simulink model "VarLoad"  (R2016a)
settings: Solver=ode23t  StartTime=0.0  StopTime=6  FixedStep=t_PWM/10  MaxStep=2e-6  RelTol=2e-4
values from neighbouring files (symbols this model uses):
  C1 = t_PWM * (N*Impp)*0.1/ (8 * (N*Vmpp)*0.0001)    [SolarPanelModel.m]
  C2 = (N*Vo) * t_PWM/ (Load * (N*Vo)*0.001)    [SolarPanelModel.m]
  Isc = G/ Gr * (Iscr + miu_Isc*(Tc - Tr))    (= 9.318625)    [SolarPanelModel.m]
  k_l = k_v/10    (= 2)    [SolarPanelModel.m]
  L_inductor = (N*Vo) * t_PWM/ (4 * (N*Impp)*0.01)    [SolarPanelModel.m]
  Rs = sol(3)    [SolarPanelModel.m]
  t_PWM = 20e-6    (= 2e-05)    [SolarPanelModel.m]
libraries: powerlib x16, powerlib_extras x3, simulink x1
settings Model: Creator=frede  LastModifiedBy=frede
settings DataIOCC: LimitDataPoints=on  SaveFormat=Array
settings HardwareCC: ProdBitPerPointer=32  ProdLargestAtomicFloat=None  ProdIntDivRoundTo=Undefined  ProdEndianess=Unspecified  ProdWordSize=32  ProdHWDeviceType=32-bit Generic
settings ModelReferenceCC: PropagateSignalLabelsOutOfModel=off
settings ConfigComp: CovModelRefEnable=Off

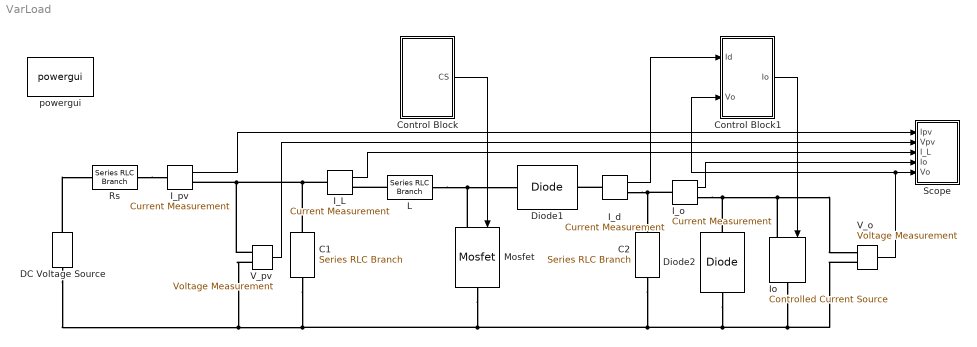
== system VarLoad ==
  C1 : powerlib/Elements/Series RLC Branch  LConnTagsString=__new0  RConnTagsString=__new0  BranchType=C  Resistance=Rs  Inductance=1e-3  SetiL0=off  InitialCurrent=0  Capacitance=C1  Setx0=off  InitialVoltage=0  Measurements=None
  C2 : powerlib/Elements/Series RLC Branch  LConnTagsString=__new0  RConnTagsString=__new0  BranchType=C  Resistance=Rs  Inductance=1e-3  SetiL0=off  InitialCurrent=0  Capacitance=C2  Setx0=off  InitialVoltage=0  Measurements=None
  Control Block : Subsystem
  Control Block1 : Subsystem
  DC Voltage Source : powerlib/Electrical Sources/DC Voltage Source  Amplitude=35  Measurements=None
  Diode1 : powerlib/Power Electronics/Diode  Ron=0.001  Lon=0  Vf=0.001  IC=0  UseSnubber=off  Rs=500  Cs=2e-9  Measurements=off
  Diode2 : powerlib/Power Electronics/Diode  Ron=0.001  Lon=0  Vf=0.001  IC=0  UseSnubber=off  Rs=500  Cs=2e-9  Measurements=off
  I_L : powerlib/Measurements/Current Measurement  PhasorSimulation=off  OutputType=Complex  PSBequivalent=0
  I_d : powerlib/Measurements/Current Measurement  PhasorSimulation=off  OutputType=Complex  PSBequivalent=0
  I_o : powerlib/Measurements/Current Measurement  PhasorSimulation=off  OutputType=Complex  PSBequivalent=0
  I_pv : powerlib/Measurements/Current Measurement  PhasorSimulation=off  OutputType=Complex  PSBequivalent=0
  Io : powerlib/Electrical Sources/Controlled Current Source  Initialize=on  Source_Type=AC  Amplitude=0  Phase=0  Frequency=0  Measurements=None
  L : powerlib/Elements/Series RLC Branch  LConnTagsString=__new0  RConnTagsString=__new0  BranchType=L  Resistance=Rs  Inductance=L_inductor  SetiL0=off  InitialCurrent=0  Capacitance=1e-6  Setx0=off  InitialVoltage=0  Measurements=None
  Mosfet : powerlib/Power Electronics/Mosfet  Ron=0.001  Lon=0  Rd=0.001  Vfd=0  IC=0  Rs=1e3  Cs=1e-7  Measurements=off
  Rs : powerlib/Elements/Series RLC Branch  LConnTagsString=__new0  RConnTagsString=__new0  BranchType=R  Resistance=0.1  Inductance=1e-3  SetiL0=off  InitialCurrent=0  Capacitance=1e-6  Setx0=off  InitialVoltage=0  Measurements=None
  Scope : Subsystem
  V_o : powerlib/Measurements/Voltage Measurement  PhasorSimulation=off  OutputType=Complex  PSBequivalent=0
  V_pv : powerlib/Measurements/Voltage Measurement  PhasorSimulation=off  OutputType=Complex  PSBequivalent=0
  powergui : powerlib/powergui  Priority=1  SimulationMode=Discrete  SolverType=Tustin/Backward Euler (TBE)  SampleTime=t_PWM/10  frequency=60  SPID=off  DisableSnubberDevices=off  DisableRonSwitches=off  DisableVfSwitches=off  SwTol=0  DisplayEquations=off  Interpol=off  ExternalGateDelay=off  methode=off  Ts=10  FunctionMessages=off  echomessages=off  HookPort=off  EnableUseOfTLC=off  x0status=blocks  frequencyindice=0  Pbase=100e6  ErrMax=1e-4  Iterations=50  UnitsV=kV  UnitsW=MW  buscounter=0  RestoreLinks=warning  ResistiveCurrentMeasurement=off  Frange=[0:2:500]  Ylog=off  Xlog=on  ShowGrid=off  save=off  variable=ZData  structure=0  ZoomFFT=off  StartTime=0.0  cycles=1  DisplayStyle=1  fundamental=60  FreqAxis=off  MaxFrequency=1000  frequencyindicesteady=1  RmsSteady=1  display=off
  wires:
  I_pv/1 -> Scope/1(Ipv)
  I_o/1 -> Scope/4(Io)
  V_o/1 -> Scope/5(Vo), Control Block1/2(Vo)
  Control Block/1(CS) -> Mosfet/1
  V_pv/1 -> Scope/2(Vpv)
  I_L/1 -> Scope/3(I_L)
  Control Block1/1(Io) -> Io/1
  I_d/1 -> Control Block1/1(Id)
  connections:
  C1/RConn1 -- DC Voltage Source/LConn1 -- V_pv/LConn2 -- Io/RConn1 -- V_o/LConn2 -- Diode2/LConn1 -- C2/RConn1 -- Mosfet/RConn1
  V_pv/LConn1 -- I_L/LConn1 -- C1/LConn1 -- I_pv/RConn1
  Mosfet/LConn1 -- L/RConn1 -- Diode1/LConn1
  I_o/LConn1 -- I_d/RConn1 -- C2/LConn1
  I_o/RConn1 -- V_o/LConn1 -- Io/LConn1 -- Diode2/RConn1
  L/LConn1 -- I_L/RConn1
  DC Voltage Source/RConn1 -- Rs/LConn1
  Rs/RConn1 -- I_pv/LConn1
  I_d/LConn1 -- Diode1/RConn1

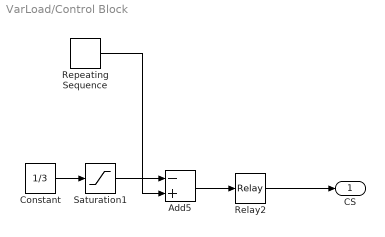
== system VarLoad/Control Block ==
  Add5 : Sum  Inputs=-+
  Constant : Constant  Value=1/3
  Relay2 : Relay  OnSwitchValue=0.0001  OffSwitchValue=-0.0001  ZeroCross=off
  Repeating Sequence : simulink/Sources/Repeating Sequence  rep_seq_t=[0 1e-4]  rep_seq_y=[0 1]
  Saturation1 : Saturate  UpperLimit=0.99  LowerLimit=0.01  ZeroCross=off
  CS : Outport
  wires:
  Relay2/1 -> CS/1
  Repeating Sequence/1 -> Add5/2
  Saturation1/1 -> Add5/1
  Add5/1 -> Relay2/1
  Constant/1 -> Saturation1/1

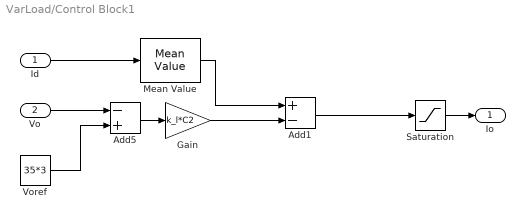
== system VarLoad/Control Block1 ==
  Id : Inport
  Vo : Inport  Port=2
  Add1 : Sum  Inputs=+-
  Add5 : Sum  Inputs=-+
  Gain : Gain  Gain=k_l*C2
  Mean Value : powerlib_extras/Measurements/Mean Value  Period=1/1000
  Saturation : Saturate  UpperLimit=Isc  LowerLimit=0
  Voref : Constant  Value=35*3
  Io : Outport
  wires:
  Vo/1 -> Add5/1
  Voref/1 -> Add5/2
  Add5/1 -> Gain/1
  Id/1 -> Mean Value/1
  Gain/1 -> Add1/2
  Add1/1 -> Saturation/1
  Saturation/1 -> Io/1
  Mean Value/1 -> Add1/1

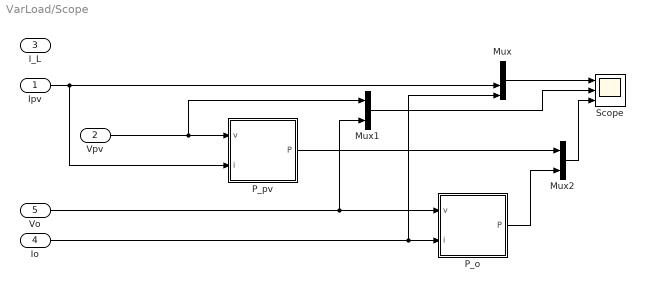
== system VarLoad/Scope ==
  Ipv : Inport
  Vpv : Inport  Port=2
  I_L : Inport  Port=3
  Io : Inport  Port=4
  Vo : Inport  Port=5
  Mux : Mux
  Mux1 : Mux  Inputs=2
  Mux2 : Mux  Inputs=2
  P_o : Subsystem
  P_pv : Subsystem
  Scope : Scope  NumInputPorts=3
  wires:
  Mux/1 -> Scope/1
  P_o/1(P) -> Mux2/2
  Mux2/1 -> Scope/3
  P_pv/1(P) -> Mux2/1
  Io/1 -> P_o/2(i), Mux/4
  Mux1/1 -> Scope/2
  Vo/1 -> P_o/1(v), Mux1/2
  Ipv/1 -> Mux/3, P_pv/2(i)
  Vpv/1 -> P_pv/1(v), Mux1/1

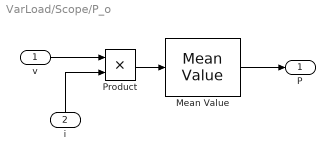
== system VarLoad/Scope/P_o ==
  v : Inport
  i : Inport  Port=2
  Mean Value : powerlib_extras/Measurements/Mean Value  Period=1/1000
  Product : Product
  P : Outport
  wires:
  Mean Value/1 -> P/1
  Product/1 -> Mean Value/1
  v/1 -> Product/1
  i/1 -> Product/2

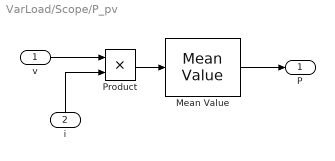
== system VarLoad/Scope/P_pv ==
  v : Inport
  i : Inport  Port=2
  Mean Value : powerlib_extras/Measurements/Mean Value  Period=1/1000
  Product : Product
  P : Outport
  wires:
  Mean Value/1 -> P/1
  Product/1 -> Mean Value/1
  v/1 -> Product/1
  i/1 -> Product/2
